simulink subsystem "navPreProcessing"  (R2026a)
settings: Solver=VariableStepAuto
values from neighbouring files (symbols this model uses):
  navControl = 1    [navParams.sldd]
settings Model: Creator=maxhu  LastModifiedBy=maxhu

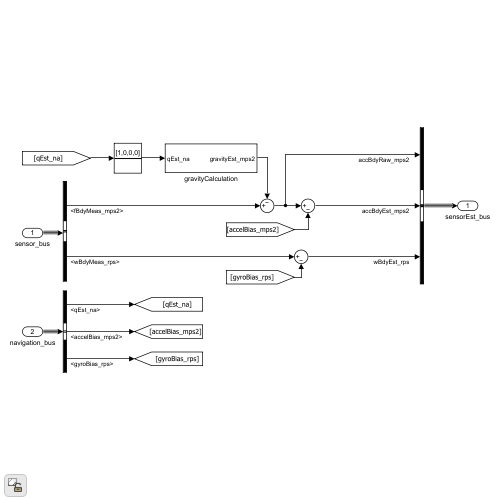
[thumbnail: Simulink's stored preview of the top-level diagram]
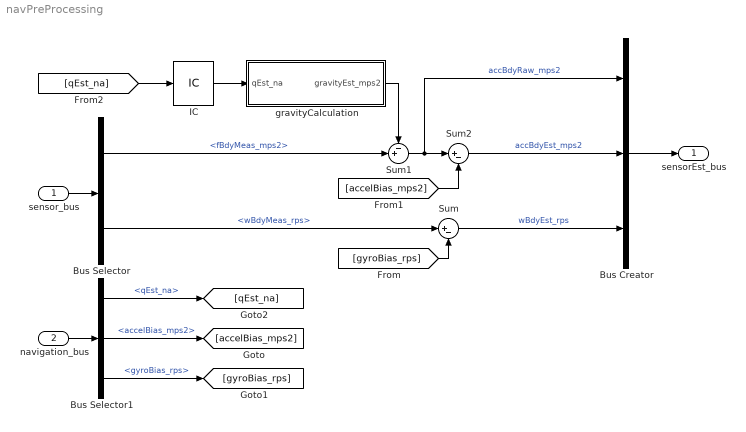
== system navPreProcessing ==
  sensor_bus : Inport
  navigation_bus : Inport  Port=2
  Bus Creator : BusCreator  Inputs=3
  Bus Selector : BusSelector  OutputSignals=fBdyMeas_mps2,wBdyMeas_rps
  Bus Selector1 : BusSelector  OutputSignals=qEst_na,accelBias_mps2,gyroBias_rps
  IC : InitialCondition  Value=[1,0,0,0]
  Sum : Sum  Inputs=|+-
  Sum1 : Sum  Inputs=-+|
  Sum2 : Sum  Inputs=|+-
  gravityCalculation : Subsystem
  sensorEst_bus : Outport
  wires:
  Sum/1 -> Bus Creator/3  "wBdyEst_rps"
  Bus Creator/1 -> sensorEst_bus/1
  Bus Selector/2 -> Sum/1  "<wBdyMeas_rps>"
  sensor_bus/1 -> Bus Selector/1
  navigation_bus/1 -> Bus Selector1/1
  Bus Selector1/2 -> [accelBias_mps2]  "<accelBias_mps2>"
  Bus Selector1/3 -> [gyroBias_rps]  "<gyroBias_rps>"
  Bus Selector1/1 -> [qEst_na]  "<qEst_na>"
  Bus Selector/1 -> Sum1/2  "<fBdyMeas_mps2>"
  [qEst_na] -> IC/1
  IC/1 -> gravityCalculation/1(qEst_na)
  [gyroBias_rps] -> Sum/2
  gravityCalculation/1(gravityEst_mps2) -> Sum1/1
  Sum2/1 -> Bus Creator/2  "accBdyEst_mps2"
  [accelBias_mps2] -> Sum2/2
  Sum1/1 -> Sum2/1, Bus Creator/1  "accBdyRaw_mps2"

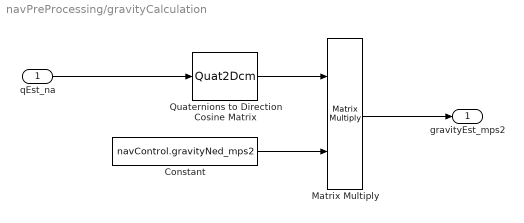
== system navPreProcessing/gravityCalculation ==
  qEst_na : Inport
  Constant : Constant  Value=navControl.gravityNed_mps2
  Matrix Multiply : Product  Multiplication=Matrix(*)
  Quaternions to Direction Cosine Matrix : Quat2Dcm
  gravityEst_mps2 : Outport
  wires:
  qEst_na/1 -> Quaternions to Direction Cosine Matrix/1
  Matrix Multiply/1 -> gravityEst_mps2/1
  Constant/1 -> Matrix Multiply/2
  Quaternions to Direction Cosine Matrix/1 -> Matrix Multiply/1
